simulink model "closedLoop_DesignTest"  (R2019b)
settings: Solver=VariableStepAuto  StartTime=0.0  StopTime=30  RelTol=1e-3
values from neighbouring files (symbols this model uses):
  A = [-0.5355 -25.1019 -6.2361;1 0 0; 0 1 0]    [testClosedLoop_Design.m]    (also in testClosedLoop_Production.m)
  A_obs = A - L*C    [testClosedLoop_Design.m]    (also in testClosedLoop_Production.m)
  B = [1 0 0]'    [testClosedLoop_Design.m]    (also in testClosedLoop_Production.m)
  B_obs = [L B - (L*D)]    [testClosedLoop_Design.m]    (also in testClosedLoop_Production.m)
  C = [0.1336 -2.2550 52.2390]    [testClosedLoop_Design.m]    (also in testClosedLoop_Production.m)
  C_obs = eye(size(A_obs))    [testClosedLoop_Design.m]    (also in testClosedLoop_Production.m)
  D = 0    [testClosedLoop_Design.m]    (also in testClosedLoop_Production.m)
  D_obs = zeros(size(B_obs))    [testClosedLoop_Design.m]    (also in testClosedLoop_Production.m)
  xhat_init = zeros(n,1)    [testClosedLoop_Design.m]    (also in testClosedLoop_Production.m)
  xinit = zeros(n,m)    [testClosedLoop_Design.m]    (also in testClosedLoop_Production.m)
undefined symbols (not defined in the file or in its folder): K
settings Model: Creator=trest  LastModifiedBy=trest

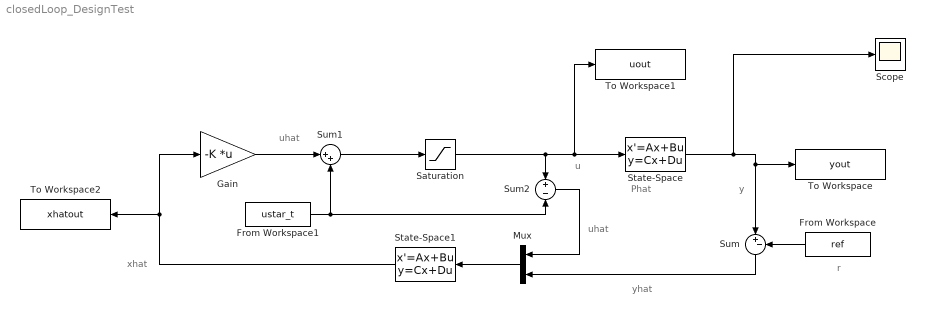
== system closedLoop_DesignTest ==
  note: uhat
  note: u
  note: xhat
  note: y
  note: yhat
  note: r
  note: uhat
  note: Phat
  From Workspace : FromWorkspace  VariableName=ref  SampleTime=0
  From Workspace1 : FromWorkspace  VariableName=ustar_t  SampleTime=0
  Gain : Gain  Gain=-K  Multiplication=Matrix(K*u)
  Mux : Mux  Inputs=2
  Saturation : Saturate  UpperLimit=5  LowerLimit=-4
  Scope : Scope
  State-Space : StateSpace  A=A  B=B  C=C  D=D  InitialCondition=xinit  ContinuousStateAttributes='plant_state'
  State-Space1 : StateSpace  A=A_obs  B=B_obs  C=C_obs  D=D_obs  InitialCondition=xhat_init  ContinuousStateAttributes='observer_state'
  Sum : Sum  Inputs=|+-
  Sum1 : Sum  Inputs=|++
  Sum2 : Sum  Inputs=+-
  To Workspace : ToWorkspace  VariableName=yout  SaveFormat=Timeseries  SampleTime=-1
  To Workspace1 : ToWorkspace  VariableName=uout  SaveFormat=Timeseries  SampleTime=-1
  To Workspace2 : ToWorkspace  VariableName=xhatout  SaveFormat=Timeseries  SampleTime=-1
  wires:
  Sum1/1 -> Saturation/1
  Mux/1 -> State-Space1/1
  Gain/1 -> Sum1/1
  Sum/1 -> Mux/2
  From Workspace/1 -> Sum/2
  Sum2/1 -> Mux/1
  Saturation/1 -> To Workspace1/1, State-Space/1, Sum2/1
  State-Space/1 -> Scope/1, To Workspace/1, Sum/1
  State-Space1/1 -> To Workspace2/1, Gain/1
  From Workspace1/1 -> Sum1/2, Sum2/2
